simulink model "tutorial10_state_feedback"  (R2025a)
settings: Solver=VariableStepAuto  StartTime=0.0  StopTime=8  RelTol=1e-3
settings Model: Creator=xing2  LastModifiedBy=xing2

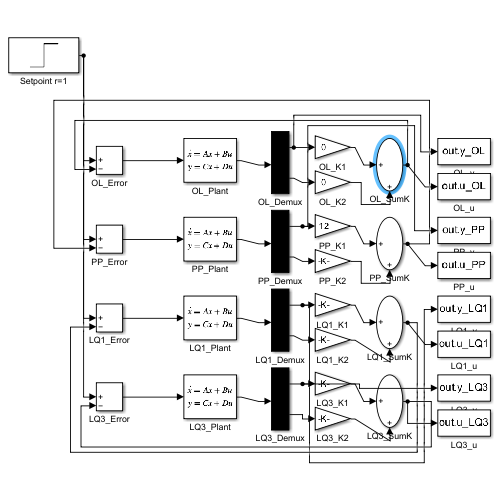
[thumbnail: Simulink's stored preview of the top-level diagram]
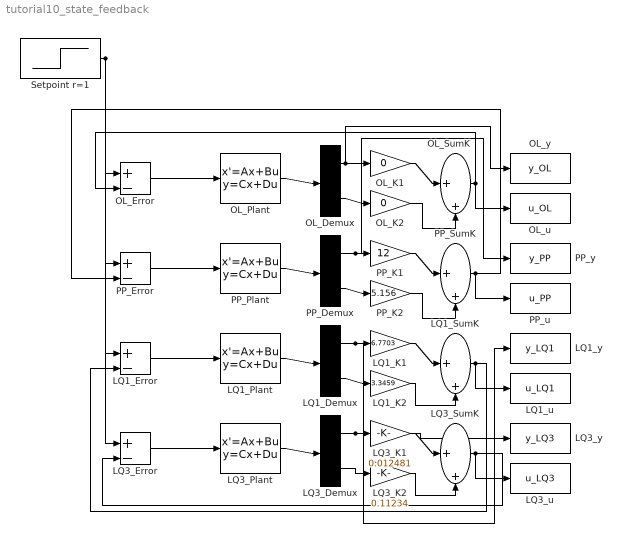
== system tutorial10_state_feedback ==
  LQ1_Demux : Demux  Outputs=2
  LQ1_Error : Sum  Inputs=|+-
  LQ1_K1 : Gain  Gain=6.7703
  LQ1_K2 : Gain  Gain=3.3459
  LQ1_Plant : StateSpace  A=[0 1;-4 -0.5]  B=[0;1]  C=eye(2)  D=zeros(2,1)  InitialCondition=[0; 0]
  LQ1_SumK : Sum  Inputs=|++
  LQ1_u : ToWorkspace  VariableName=u_LQ1  SaveFormat=Timeseries  SampleTime=-1
  LQ1_y : ToWorkspace  VariableName=y_LQ1  SaveFormat=Timeseries  SampleTime=-1
  LQ3_Demux : Demux  Outputs=2
  LQ3_Error : Sum  Inputs=|+-
  LQ3_K1 : Gain  Gain=0.012481
  LQ3_K2 : Gain  Gain=0.11234
  LQ3_Plant : StateSpace  A=[0 1;-4 -0.5]  B=[0;1]  C=eye(2)  D=zeros(2,1)  InitialCondition=[0; 0]
  LQ3_SumK : Sum  Inputs=|++
  LQ3_u : ToWorkspace  VariableName=u_LQ3  SaveFormat=Timeseries  SampleTime=-1
  LQ3_y : ToWorkspace  VariableName=y_LQ3  SaveFormat=Timeseries  SampleTime=-1
  OL_Demux : Demux  Outputs=2
  OL_Error : Sum  Inputs=|+-
  OL_K1 : Gain  Gain=0
  OL_K2 : Gain  Gain=0
  OL_Plant : StateSpace  A=[0 1;-4 -0.5]  B=[0;1]  C=eye(2)  D=zeros(2,1)  InitialCondition=[0; 0]
  OL_SumK : Sum  Inputs=|++
  OL_u : ToWorkspace  VariableName=u_OL  SaveFormat=Timeseries  SampleTime=-1
  OL_y : ToWorkspace  VariableName=y_OL  SaveFormat=Timeseries  SampleTime=-1
  PP_Demux : Demux  Outputs=2
  PP_Error : Sum  Inputs=|+-
  PP_K1 : Gain  Gain=12
  PP_K2 : Gain  Gain=5.156
  PP_Plant : StateSpace  A=[0 1;-4 -0.5]  B=[0;1]  C=eye(2)  D=zeros(2,1)  InitialCondition=[0; 0]
  PP_SumK : Sum  Inputs=|++
  PP_u : ToWorkspace  VariableName=u_PP  SaveFormat=Timeseries  SampleTime=-1
  PP_y : ToWorkspace  VariableName=y_PP  SaveFormat=Timeseries  SampleTime=-1
  Setpoint r=1 : Step  Time=0.5  SampleTime=0
  wires:
  Setpoint r=1/1 -> OL_Error/1, PP_Error/1, LQ1_Error/1, LQ3_Error/1
  OL_Error/1 -> OL_Plant/1
  OL_Plant/1 -> OL_Demux/1
  OL_Demux/1 -> OL_K1/1, OL_y/1
  OL_Demux/2 -> OL_K2/1
  OL_K1/1 -> OL_SumK/1
  OL_K2/1 -> OL_SumK/2
  OL_SumK/1 -> OL_Error/2, OL_u/1
  PP_Error/1 -> PP_Plant/1
  PP_Plant/1 -> PP_Demux/1
  PP_Demux/1 -> PP_K1/1, PP_y/1
  PP_Demux/2 -> PP_K2/1
  PP_K1/1 -> PP_SumK/1
  PP_K2/1 -> PP_SumK/2
  PP_SumK/1 -> PP_Error/2, PP_u/1
  LQ1_Error/1 -> LQ1_Plant/1
  LQ1_Plant/1 -> LQ1_Demux/1
  LQ1_Demux/1 -> LQ1_K1/1, LQ1_y/1
  LQ1_Demux/2 -> LQ1_K2/1
  LQ1_K1/1 -> LQ1_SumK/1
  LQ1_K2/1 -> LQ1_SumK/2
  LQ1_SumK/1 -> LQ1_Error/2, LQ1_u/1
  LQ3_Error/1 -> LQ3_Plant/1
  LQ3_Plant/1 -> LQ3_Demux/1
  LQ3_Demux/1 -> LQ3_K1/1, LQ3_y/1
  LQ3_Demux/2 -> LQ3_K2/1
  LQ3_K1/1 -> LQ3_SumK/1
  LQ3_K2/1 -> LQ3_SumK/2
  LQ3_SumK/1 -> LQ3_Error/2, LQ3_u/1
